simulink library "hvs_framelib_bevlh_det_emot"  (R2016a)
settings: Solver=ode1  StartTime=0.0  StopTime=Inf  FixedStep=0.001  RelTol=1e-3
undefined symbols (not defined in the file): aux_power_flag, dcdc_effmap, dcdc_effmap_cooltemp_3rdD, dcdc_effmap_cur_2ndD, dcdc_effmap_vlt_1stD
libraries: Electrical_to_Mechanical_gen x6, Electrical_converter x4, Electrical_to_Thermal_gen x2, Electrical_charger x2, Powernet x2, Enrg_conv_El_to_Mec_Bosch x2, ePTO x2, simulink x2
(part 2 of 2)

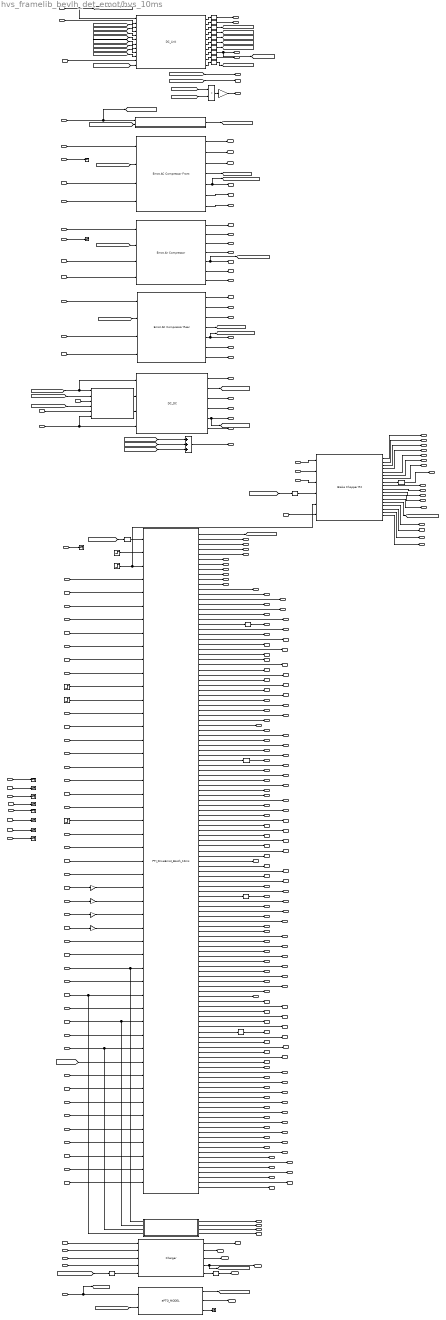
== system hvs_framelib_bevlh_det_emot/hvs_10ms ==
  hvs_dcLink_electricalEnergyStorage_voltage : Inport
  hvs_dcLink_ControllableEnergySource_current : Inport  Port=2
  hvs_dcdcConverter_current : Inport  Port=3
  hvs_driveInverter_coolant_temperature : Inport  Port=4
  hvs_drvEmot1Oil_Temperature : Inport  Port=5
  hvs_brakeResistor_coolant_temperature : Inport  Port=6
  hvs_auxPowerInverter_coolant_temperature : Inport  Port=7
  hvs_inverterAirCompressor_coolant_temperature : Inport  Port=8
  hvs_emot_Emot1_angPos : Inport  Port=9
  hvs_emot_Emot1_angVel : Inport  Port=10
  hvs_emot_Emot1_angAcc : Inport  Port=11
  hvs_emot_Emot2_angAcc : Inport  Port=12
  hvs_emot_Emot2_angPos : Inport  Port=13
  hvs_emot_Emot2_angVel : Inport  Port=14
  hvs_emot_Emot3_angAcc : Inport  Port=15
  hvs_emot_Emot3_angPos : Inport  Port=16
  hvs_emot_Emot3_angVel : Inport  Port=17
  hvs_emot_Emot4_angAcc : Inport  Port=18
  hvs_emot_Emot4_angPos : Inport  Port=19
  hvs_emot_Emot4_angVel : Inport  Port=20
  hvs_emot_AirCompressor_torque : Inport  Port=21
  brc_ControlMode : Inport  Port=22
  brc_PowerReqCh1_kW : Inport  Port=23
  brc_PowerReqCh2_kW : Inport  Port=24
  edcu_EMD1_CMD_ClearErrors : Inport  Port=25
  edcu_EMD1_CMD_ControlMode : Inport  Port=26
  edcu_EMD1_CMD_SpeedRefLim : Inport  Port=27
  pti_tqDesired_PTI1 : Inport  Port=28
  edcu_EMD4_CMD_ClearErrors : Inport  Port=29
  edcu_EMD4_CMD_ControlMode : Inport  Port=30
  edcu_EMD4_CMD_SpeedRefLim : Inport  Port=31
  pti_tqDesired_PTI4 : Inport  Port=32
  vccu_PlugChrg_Stat : Inport  Port=33
  vccu_Pwr_ChargSysSoll : Inport  Port=34
  vccu_TestPwrSLQ_Out : Inport  Port=35
  vccu_CAN_MaxPlginChrgPwrLim : Inport  Port=36
  hvs_emot_AirCondFrontHV_torque : Inport  Port=37
  hvs_emot_AirCondRearHV_torque : Inport  Port=38
  hvsAux_InverterAirCompressor_torque_Rq : Inport  Port=39
  hvsAux_InverterAirCompressor_Voltage_Rq : Inport  Port=40
  hvsAux_InverterAcCompressorFront_torque_Rq : Inport  Port=41
  hvsAux_InverterAcCompressorFront_Voltage_Rq : Inport  Port=42
  hvsAux_InverterAcCompressorRear_torque_Rq : Inport  Port=43
  hvsAux_InverterAcCompressorRear_Voltage_Rq : Inport  Port=44
  hvsAux_dcdcConverter_LvVoltage_Rq : Inport  Port=45
  env_dcLink_aux_power : Inport  Port=46
  edcu_EMD2_CMD_ClearErrors : Inport  Port=47
  edcu_EMD2_CMD_ControlMode : Inport  Port=48
  edcu_EMD2_CMD_SpeedRefLim : Inport  Port=49
  pti_tqDesired_PTI2 : Inport  Port=50
  edcu_EMD3_CMD_ClearErrors : Inport  Port=51
  edcu_EMD3_CMD_ControlMode : Inport  Port=52
  edcu_EMD3_CMD_SpeedRefLim : Inport  Port=53
  pti_tqDesired_PTI3 : Inport  Port=54
  hvs_DCBoxCoolant_Temperature : Inport  Port=55
  hvs_coolHV_current : Inport  Port=56
  env_Temperature : Inport  Port=57
  hvs_drvEmotCoolant_Temperature : Inport  Port=58
  hvs_drvEmot4Oil_Temperature : Inport  Port=59
  hvs_drvEmot2Oil_Temperature : Inport  Port=60
  hvs_drvEmot3Oil_Temperature : Inport  Port=61
  hvs_drvEmot1Coolant_Temperature : Inport  Port=62
  hvs_drvEmot2Coolant_Temperature : Inport  Port=63
  hvs_drvEmot3Coolant_Temperature : Inport  Port=64
  hvs_drvEmot4Coolant_Temperature : Inport  Port=65
  pti_frqSwt_PTI1 : Inport  Port=66
  pti_frqSwt_PTI2 : Inport  Port=67
  pti_frqSwt_PTI3 : Inport  Port=68
  pti_frqSwt_PTI4 : Inport  Port=69
  hvs_drvEmot1CoolantFlow_vdot : Inport  Port=70
  hvs_drvEmot1OilFlow_vdot : Inport  Port=71
  hvs_driveInverterCoolantFlow_vdot : Inport  Port=72
  hvs_drvEmot4CoolantFlow_vdot : Inport  Port=73
  hvs_drvEmot4OilFlow_vdot : Inport  Port=74
  hvs_drvEmot2CoolantFlow_vdot : Inport  Port=75
  hvs_drvEmot2OilFlow_vdot : Inport  Port=76
  hvs_drvEmot3CoolantFlow_vdot : Inport  Port=77
  hvs_drvEmot3OilFlow_vdot : Inport  Port=78
  Brake Chopper RX1 : Electrical_to_Thermal_gen/Brake Chopper RX
  Charger : Electrical_charger/Charger
  DC_DC : Electrical_converter/DC_DC
  DC_Link : Powernet/DC_Link
  EDCU_Dig_SafetyCutOffDG1 : Step  Time=0.812
  Emot AC Compressor Front Generic : Electrical_to_Mechanical_gen/Emot AC Compressor Front
  Emot AC Compressor Rear Generic : Electrical_to_Mechanical_gen/Emot AC Compressor Rear
  Emot Air Compressor Generic : Electrical_to_Mechanical_gen/Emot Air Compressor
  Gain7 : Gain  Gain=1/1000
  HVFreigabeHW1_SiRelay_D : Step  Time=5.502
  HVFreigabeHW2_SiRelay_D : Step  Time=5.502
  HVFreigabeHW3_SiRelay_D : Step  Time=5.502
  HVFreigabeHW4_SiRelay_D : Step  Time=5.502
  PTI_DriveEmot_Bosch_10ms : Enrg_conv_El_to_Mec_Bosch/PTI_DriveEmot_Bosch_10ms
  Process : Subsystem
  Product2 : Product  Inputs=**  RndMeth=Zero
  Rename_Signals_for_PTI_detailed : Subsystem
  Reshape{,1..18} (19 alike) : Reshape
  Sum8 : Sum  Inputs=+++  SaturateOnIntegerOverflow=on  InputSameDT=on  OutDataTypeStr=Inherit: Same as first input
  Terminator{,1..10,15} (12 alike) : Terminator
  ePTO_MODEL : ePTO/ePTO_MODEL
  rad/sectorpm{,1..3} (4 alike) : Gain  Gain=30/pi
  sub_env_aux : Subsystem
  hvs_dcLink_electricalEnergyStorage_current : Outport
  hvs_dcLink_ControllableEnergySource_voltage : Outport  Port=2
  hvs_dcdcConverter_voltage : Outport  Port=3
  hvs_driveInverter_wasteHeat_power : Outport  Port=4
  hvs_drvEmotWasteHeat_power : Outport  Port=5
  hvs_drvEmot1WasteHeat_power : Outport  Port=6
  hvs_drvEmot2WasteHeat_power : Outport  Port=7
  hvs_drvEmot3WasteHeat_power : Outport  Port=8
  hvs_drvEmot4WasteHeat_power : Outport  Port=9
  hvs_brakeResistor_wasteHeat_power : Outport  Port=10
  hvs_auxPowerInverter_wasteHeat_power : Outport  Port=11
  hvs_inverterAirCompressor_wasteHeat_power : Outport  Port=12
  hvs_emot_Emot1_torque : Outport  Port=13
  hvs_emot_Emot2_torque : Outport  Port=14
  hvs_emot_Emot3_torque : Outport  Port=15
  hvs_emot_Emot4_torque : Outport  Port=16
  hvs_emot_AirCompressor_angAcc : Outport  Port=17
  hvs_emot_AirCompressor_angPos : Outport  Port=18
  hvs_emot_AirCompressor_angVel : Outport  Port=19
  hvs_emot_AirCondFrontHV_angAcc : Outport  Port=20
  hvs_emot_AirCondFrontHV_angPos : Outport  Port=21
  hvs_emot_AirCondFrontHV_angVel : Outport  Port=22
  hvs_emot_AirCondRearHV_angAcc : Outport  Port=23
  hvs_emot_AirCondRearHV_angVel : Outport  Port=24
  hvs_emot_AirCondRearHV_angPos : Outport  Port=25
  hvs_BRC_ACT_DigitalInput1 : Outport  Port=26
  hvs_BRC_ACT_InverterState : Outport  Port=27
  hvs_BRC_ACT_MaxAvailablePowerCh1 : Outport  Port=28
  hvs_BRC_ACT_MaxAvailablePowerCh1_VAL : Outport  Port=29
  hvs_BRC_ACT_PowerCh1 : Outport  Port=30
  hvs_BRC_ACT_MaxAvailablePowerCh2 : Outport  Port=31
  hvs_BRC_ACT_PowerCh2 : Outport  Port=32
  hvs_BRC_ACT_DcLinkVoltage : Outport  Port=33
  hvs_BRC_ACT_ExtTemperatureCh1 : Outport  Port=34
  hvs_BRC_ACT_ExtTemperatureCh2 : Outport  Port=35
  hvs_BRC_ACT_JunctionTempCh1 : Outport  Port=36
  hvs_BRC_ACT_JunctionTempCh2 : Outport  Port=37
  hvs_EMD1_ACT_DigitalInput1 : Outport  Port=38
  hvs_EMD1_ACT_InverterState : Outport  Port=39
  hvs_EMD1_ACT_MaxAvailableTorque : Outport  Port=40
  hvs_EMD1_ACT_ReferenceTorqueLim : Outport  Port=41
  hvs_EMD1_ACT_Torque : Outport  Port=42
  hvs_EMD1_ACT_DcLinkPower : Outport  Port=43
  hvs_EMD1_ACT_MotorSpeed : Outport  Port=44
  hvs_EMD1_ACT_DcLinkVoltage : Outport  Port=45
  hvs_EMD1_ACT_MaxJunctionTemp : Outport  Port=46
  hvs_EMD1_ACT_MotorTemperature : Outport  Port=47
  hvs_EMD1_ACT_RotorTemperature : Outport  Port=48
  hvs_EMD1_ACT_InverterLosses : Outport  Port=49
  hvs_EMD1_ACT_MotorLosses : Outport  Port=50
  hvs_EMD1_uStator : Outport  Port=51
  hvs_EMD1_iStator : Outport  Port=52
  hvs_EMD1_modIdx : Outport  Port=53
  hvs_EMD1_cosPhi : Outport  Port=54
  hvs_EMD1_ACT_tSnsrPwrModlMax : Outport  Port=55
  hvs_EMD1_ACT_tCapSnsr : Outport  Port=56
  hvs_EMD1_ACT_tCapCoil : Outport  Port=57
  hvs_EMD1_ACT_tCapAcCnctr : Outport  Port=58
  hvs_EMD1_ACT_tCapDcCnctr : Outport  Port=59
  hvs_EMD1_ACT_tIvtrAcRail : Outport  Port=60
  hvs_EMD1_ACT_tIvtrDcRail : Outport  Port=61
  hvs_EMD1_ACT_tIvtrAcRailIphaSnsr : Outport  Port=62
  hvs_EMD1_ACT_tIvtrDcRailCnctr : Outport  Port=63
  hvs_EMD1_ACT_tCoolIvtrOuttk : Outport  Port=64
  hvs_EMD1_ACT_tCoolantIvtrIntk : Outport  Port=65
  hvs_EMD4_ACT_DigitalInput1 : Outport  Port=66
  hvs_EMD4_ACT_InverterState : Outport  Port=67
  hvs_EMD4_ACT_MaxAvailableTorque : Outport  Port=68
  hvs_EMD4_ACT_ReferenceTorqueLim : Outport  Port=69
  hvs_EMD4_ACT_Torque : Outport  Port=70
  hvs_EMD4_ACT_DcLinkPower : Outport  Port=71
  hvs_EMD4_ACT_MotorSpeed : Outport  Port=72
  hvs_EMD4_ACT_DcLinkVoltage : Outport  Port=73
  hvs_EMD4_ACT_MaxJunctionTemperature : Outport  Port=74
  hvs_EMD4_ACT_MotorTemperature : Outport  Port=75
  hvs_EMD4_ACT_RotorTemperature : Outport  Port=76
  hvs_EMD4_ACT_InverterLosses : Outport  Port=77
  hvs_EMD4_ACT_MotorLosses : Outport  Port=78
  hvs_EMD4_uStator : Outport  Port=79
  hvs_EMD4_iStator : Outport  Port=80
  hvs_EMD4_modIdx : Outport  Port=81
  hvs_EMD4_cosPhi : Outport  Port=82
  hvs_EMD4_ACT_tSnsrPwrModlMax : Outport  Port=83
  hvs_EMD4_ACT_tCapSnsr : Outport  Port=84
  hvs_EMD4_ACT_tCapCoil : Outport  Port=85
  hvs_EMD4_ACT_tCapAcCnctr : Outport  Port=86
  hvs_EMD4_ACT_tCapDcCnctr : Outport  Port=87
  hvs_EMD4_ACT_tIvtrAcRail : Outport  Port=88
  hvs_EMD4_ACT_tIvtrDcRail : Outport  Port=89
  hvs_EMD4_ACT_tIvtrAcRailIphaSnsr : Outport  Port=90
  hvs_EMD4_ACT_tIvtrDcRailCnctr : Outport  Port=91
  hvs_EMD4_ACT_tCoolIvtrOuttk : Outport  Port=92
  hvs_EMD4_ACT_tCoolantIvtrIntk : Outport  Port=93
  hvs_EMD3_ACT_DigitalInput1 : Outport  Port=94
  hvs_EMD3_ACT_InverterState : Outport  Port=95
  hvs_EMD3_ACT_MaxAvailableTorque : Outport  Port=96
  hvs_EMD3_ACT_ReferenceTorqueLim : Outport  Port=97
  hvs_EMD3_ACT_Torque : Outport  Port=98
  hvs_EMD3_ACT_DcLinkPower : Outport  Port=99
  hvs_EMD3_ACT_MotorSpeed : Outport  Port=100
  hvs_EMD3_ACT_DcLinkVoltage : Outport  Port=101
  hvs_EMD3_ACT_MaxJunctionTemp : Outport  Port=102
  hvs_EMD3_ACT_MotorTemperature : Outport  Port=103
  hvs_EMD3_ACT_RotorTemperature : Outport  Port=104
  hvs_EMD3_ACT_InverterLosses : Outport  Port=105
  hvs_EMD3_ACT_MotorLosses : Outport  Port=106
  hvs_EMD3_uStator : Outport  Port=107
  hvs_EMD3_iStator : Outport  Port=108
  hvs_EMD3_modIdx : Outport  Port=109
  hvs_EMD3_cosPhi : Outport  Port=110
  hvs_EMD3_ACT_tSnsrPwrModlMax : Outport  Port=111
  hvs_EMD3_ACT_tCapSnsr : Outport  Port=112
  hvs_EMD3_ACT_tCapCoil : Outport  Port=113
  hvs_EMD3_ACT_tCapAcCnctr : Outport  Port=114
  hvs_EMD3_ACT_tCapDcCnctr : Outport  Port=115
  hvs_EMD3_ACT_tIvtrAcRail : Outport  Port=116
  hvs_EMD3_ACT_tIvtrDcRail : Outport  Port=117
  hvs_EMD3_ACT_tIvtrAcRailIphaSnsr : Outport  Port=118
  hvs_EMD3_ACT_tIvtrDcRailCnctr : Outport  Port=119
  hvs_EMD3_ACT_tCoolIvtrOuttk : Outport  Port=120
  hvs_EMD3_ACT_tCoolantIvtrIntk : Outport  Port=121
  hvs_EMD2_ACT_DigitalInput1 : Outport  Port=122
  hvs_EMD2_ACT_InverterState : Outport  Port=123
  hvs_EMD2_ACT_MaxAvailableTorque : Outport  Port=124
  hvs_EMD2_ACT_ReferenceTorqueLim : Outport  Port=125
  hvs_EMD2_ACT_Torque : Outport  Port=126
  hvs_EMD2_ACT_DcLinkPower : Outport  Port=127
  hvs_EMD2_ACT_MotorSpeed : Outport  Port=128
  hvs_EMD2_ACT_DcLinkVoltage : Outport  Port=129
  hvs_EMD2_ACT_MaxJunctionTemp : Outport  Port=130
  hvs_EMD2_ACT_MotorTemperature : Outport  Port=131
  hvs_EMD2_ACT_RotorTemperature : Outport  Port=132
  hvs_EMD2_ACT_InverterLosses : Outport  Port=133
  hvs_EMD2_ACT_MotorLosses : Outport  Port=134
  hvs_EMD2_uStator : Outport  Port=135
  hvs_EMD2_iStator : Outport  Port=136
  hvs_EMD2_modIdx : Outport  Port=137
  hvs_EMD2_cosPhi : Outport  Port=138
  hvs_EMD2_ACT_tSnsrPwrModlMax : Outport  Port=139
  hvs_EMD2_ACT_tCapSnsr : Outport  Port=140
  hvs_EMD2_ACT_tCapCoil : Outport  Port=141
  hvs_EMD2_ACT_tCapAcCnctr : Outport  Port=142
  hvs_EMD2_ACT_tCapDcCnctr : Outport  Port=143
  hvs_EMD2_ACT_tIvtrAcRail : Outport  Port=144
  hvs_EMD2_ACT_tIvtrDcRail : Outport  Port=145
  hvs_EMD2_ACT_tIvtrAcRailIphaSnsr : Outport  Port=146
  hvs_EMD2_ACT_tIvtrDcRailCnctr : Outport  Port=147
  hvs_EMD2_ACT_tCoolIvtrOuttk : Outport  Port=148
  hvs_EMD2_ACT_tCoolantIvtrIntk : Outport  Port=149
  hvs_charger_pwrChrgPhy : Outport  Port=150
  hvs_charger_ExtChrgr_Isolation_ResistanceCval : Outport  Port=151
  hvs_VCCU_DCLInk_vlt : Outport  Port=152
  hvs_InverterAirCompressor_hvCurrent : Outport  Port=153
  hvs_InverterAirCompressor_hvVoltage : Outport  Port=154
  hvs_emot_AirCompressor_nEmot : Outport  Port=155
  hvs_InverterAcCompressor_hvCurrent : Outport  Port=156
  hvs_InverterAcCompressor_hvVoltage : Outport  Port=157
  hvs_emot_AcCompressor_nEmot : Outport  Port=158
  hvs_InverterAcCompressorRear_hvCurrent : Outport  Port=159
  hvs_InverterAcCompressorRear_hvVoltage : Outport  Port=160
  hvs_emot_AcCompressorRear_nEmot : Outport  Port=161
  hvs_dcdcConverter_HvVoltage : Outport  Port=162
  hvs_dcdcConverter_LvVoltage : Outport  Port=163
  hvs_dcdcConverter_HvCurrent : Outport  Port=164
  hvs_dcdcConverter_LvCurrent : Outport  Port=165
  hvs_dcLink_aux_current : Outport  Port=166
  hvs_DCBoxWasteHeat_power : Outport  Port=167
  hvs_coolHV_voltage : Outport  Port=168
  hvs_ePTO_Elec_Power : Outport  Port=169
  hvs_charger_current : Outport  Port=170
  hvs_dcLink_drive_emot_current : Outport  Port=171
  hvs_dcLink_BrakeResistor_current : Outport  Port=172
  hvs_dcLink_aux_Power : Outport  Port=173
  hvs_EMD2_ACT_Torque_Nm : Outport  Port=174
  hvs_EMD3_ACT_Torque_Nm : Outport  Port=175
  hvs_EMD1_ACT_Torque_Nm : Outport  Port=176
  hvs_EMD4_ACT_Torque_Nm : Outport  Port=177
  hvs_drvEmot2WasteHeatcoolant_power : Outport  Port=178
  hvs_drvEmot2WasteHeatoil_power : Outport  Port=179
  hvs_drvEmot3WasteHeatcoolant_power : Outport  Port=180
  hvs_drvEmot3WasteHeatoil_power : Outport  Port=181
  hvs_drvEmot1WasteHeatcoolant_power : Outport  Port=182
  hvs_drvEmot1WasteHeatoil_power : Outport  Port=183
  hvs_drvEmot4WasteHeatcoolant_power : Outport  Port=184
  hvs_drvEmot4WasteHeatoil_power : Outport  Port=185
  hvs_BRC_ACT_MaxAvailablePowerCh1_kW : Outport  Port=186
  hvs_BRC_ACT_PowerCh1_kW : Outport  Port=187
  hvs_BRC_ACT_MaxAvailablePowerCh2_kW : Outport  Port=188
  hvs_BRC_ACT_PowerCh2_kW : Outport  Port=189
  wires:
  [hvs_dcLink_aux_current] -> Product2/1
  [hvs_APIs_DCLink_vlt] -> Product2/2
  Product2/1 -> Gain7/1
  Gain7/1 -> hvs_dcLink_aux_Power/1
  Rename_Signals_for_PTI_detailed/1(hvs_EMD1_ACT_tCoolantIvtrIntk) -> hvs_EMD1_ACT_tCoolantIvtrIntk/1
  Rename_Signals_for_PTI_detailed/4(hvs_EMD4_ACT_tCoolantIvtrIntk) -> hvs_EMD4_ACT_tCoolantIvtrIntk/1
  Rename_Signals_for_PTI_detailed/3(hvs_EMD3_ACT_tCoolantIvtrIntk) -> hvs_EMD3_ACT_tCoolantIvtrIntk/1
  Rename_Signals_for_PTI_detailed/2(hvs_EMD2_ACT_tCoolantIvtrIntk) -> hvs_EMD2_ACT_tCoolantIvtrIntk/1
  hvs_drvEmot2Coolant_Temperature/1 -> Rename_Signals_for_PTI_detailed/2(hvs_drvEmot2Coolant_Temperature), PTI_DriveEmot_Bosch_10ms/37
  PTI_DriveEmot_Bosch_10ms/27 -> hvs_EMD1_modIdx/1
  PTI_DriveEmot_Bosch_10ms/28 -> hvs_EMD1_cosPhi/1
  PTI_DriveEmot_Bosch_10ms/38 -> hvs_EMD1_ACT_tCoolIvtrOuttk/1
  PTI_DriveEmot_Bosch_10ms/37 -> hvs_EMD1_ACT_tIvtrDcRailCnctr/1
  PTI_DriveEmot_Bosch_10ms/36 -> hvs_EMD1_ACT_tIvtrAcRailIphaSnsr/1
  PTI_DriveEmot_Bosch_10ms/35 -> hvs_EMD1_ACT_tIvtrDcRail/1
  PTI_DriveEmot_Bosch_10ms/34 -> hvs_EMD1_ACT_tIvtrAcRail/1
  PTI_DriveEmot_Bosch_10ms/33 -> hvs_EMD1_ACT_tCapDcCnctr/1
  PTI_DriveEmot_Bosch_10ms/32 -> hvs_EMD1_ACT_tCapAcCnctr/1
  PTI_DriveEmot_Bosch_10ms/31 -> hvs_EMD1_ACT_tCapCoil/1
  PTI_DriveEmot_Bosch_10ms/29 -> hvs_EMD1_ACT_tSnsrPwrModlMax/1
  PTI_DriveEmot_Bosch_10ms/30 -> hvs_EMD1_ACT_tCapSnsr/1
  PTI_DriveEmot_Bosch_10ms/53 -> hvs_EMD4_iStator/1
  PTI_DriveEmot_Bosch_10ms/52 -> hvs_EMD4_uStator/1
  PTI_DriveEmot_Bosch_10ms/51 -> hvs_EMD4_ACT_MotorLosses/1
  PTI_DriveEmot_Bosch_10ms/50 -> hvs_EMD4_ACT_InverterLosses/1
  PTI_DriveEmot_Bosch_10ms/49 -> hvs_EMD4_ACT_RotorTemperature/1
  PTI_DriveEmot_Bosch_10ms/48 -> hvs_EMD4_ACT_MotorTemperature/1
  PTI_DriveEmot_Bosch_10ms/47 -> hvs_EMD4_ACT_MaxJunctionTemperature/1
  PTI_DriveEmot_Bosch_10ms/46 -> Reshape10/1
  PTI_DriveEmot_Bosch_10ms/45 -> hvs_EMD4_ACT_MotorSpeed/1
  PTI_DriveEmot_Bosch_10ms/44 -> hvs_EMD4_ACT_DcLinkPower/1
  PTI_DriveEmot_Bosch_10ms/43 -> hvs_EMD4_ACT_Torque/1
  PTI_DriveEmot_Bosch_10ms/42 -> hvs_EMD4_ACT_ReferenceTorqueLim/1
  PTI_DriveEmot_Bosch_10ms/41 -> hvs_EMD4_ACT_MaxAvailableTorque/1
  PTI_DriveEmot_Bosch_10ms/40 -> hvs_EMD4_ACT_InverterState/1
  PTI_DriveEmot_Bosch_10ms/39 -> hvs_EMD4_ACT_DigitalInput1/1
  PTI_DriveEmot_Bosch_10ms/54 -> hvs_EMD4_modIdx/1
  PTI_DriveEmot_Bosch_10ms/55 -> hvs_EMD4_cosPhi/1
  PTI_DriveEmot_Bosch_10ms/58 -> hvs_EMD4_ACT_tCapCoil/1
  PTI_DriveEmot_Bosch_10ms/59 -> hvs_EMD4_ACT_tCapAcCnctr/1
  PTI_DriveEmot_Bosch_10ms/60 -> hvs_EMD4_ACT_tCapDcCnctr/1
  PTI_DriveEmot_Bosch_10ms/61 -> hvs_EMD4_ACT_tIvtrAcRail/1
  PTI_DriveEmot_Bosch_10ms/62 -> hvs_EMD4_ACT_tIvtrDcRail/1
  PTI_DriveEmot_Bosch_10ms/63 -> hvs_EMD4_ACT_tIvtrAcRailIphaSnsr/1
  PTI_DriveEmot_Bosch_10ms/64 -> hvs_EMD4_ACT_tIvtrDcRailCnctr/1
  PTI_DriveEmot_Bosch_10ms/65 -> hvs_EMD4_ACT_tCoolIvtrOuttk/1
  PTI_DriveEmot_Bosch_10ms/56 -> hvs_EMD4_ACT_tSnsrPwrModlMax/1
  PTI_DriveEmot_Bosch_10ms/57 -> hvs_EMD4_ACT_tCapSnsr/1
  PTI_DriveEmot_Bosch_10ms/80 -> hvs_EMD3_iStator/1
  PTI_DriveEmot_Bosch_10ms/79 -> hvs_EMD3_uStator/1
  PTI_DriveEmot_Bosch_10ms/78 -> hvs_EMD3_ACT_MotorLosses/1
  PTI_DriveEmot_Bosch_10ms/77 -> hvs_EMD3_ACT_InverterLosses/1
  PTI_DriveEmot_Bosch_10ms/76 -> hvs_EMD3_ACT_RotorTemperature/1
  PTI_DriveEmot_Bosch_10ms/75 -> hvs_EMD3_ACT_MotorTemperature/1
  PTI_DriveEmot_Bosch_10ms/74 -> hvs_EMD3_ACT_MaxJunctionTemp/1
  PTI_DriveEmot_Bosch_10ms/73 -> Reshape13/1
  PTI_DriveEmot_Bosch_10ms/72 -> hvs_EMD3_ACT_MotorSpeed/1
  PTI_DriveEmot_Bosch_10ms/71 -> hvs_EMD3_ACT_DcLinkPower/1
  PTI_DriveEmot_Bosch_10ms/70 -> hvs_EMD3_ACT_Torque/1
  PTI_DriveEmot_Bosch_10ms/69 -> hvs_EMD3_ACT_ReferenceTorqueLim/1
  PTI_DriveEmot_Bosch_10ms/68 -> hvs_EMD3_ACT_MaxAvailableTorque/1
  PTI_DriveEmot_Bosch_10ms/67 -> hvs_EMD3_ACT_InverterState/1
  PTI_DriveEmot_Bosch_10ms/66 -> hvs_EMD3_ACT_DigitalInput1/1
  PTI_DriveEmot_Bosch_10ms/81 -> hvs_EMD3_modIdx/1
  PTI_DriveEmot_Bosch_10ms/82 -> hvs_EMD3_cosPhi/1
  PTI_DriveEmot_Bosch_10ms/83 -> hvs_EMD3_ACT_tSnsrPwrModlMax/1
  PTI_DriveEmot_Bosch_10ms/84 -> hvs_EMD3_ACT_tCapSnsr/1
  PTI_DriveEmot_Bosch_10ms/85 -> hvs_EMD3_ACT_tCapCoil/1
  PTI_DriveEmot_Bosch_10ms/86 -> hvs_EMD3_ACT_tCapAcCnctr/1
  PTI_DriveEmot_Bosch_10ms/87 -> hvs_EMD3_ACT_tCapDcCnctr/1
  PTI_DriveEmot_Bosch_10ms/88 -> hvs_EMD3_ACT_tIvtrAcRail/1
  PTI_DriveEmot_Bosch_10ms/89 -> hvs_EMD3_ACT_tIvtrDcRail/1
  PTI_DriveEmot_Bosch_10ms/90 -> hvs_EMD3_ACT_tIvtrAcRailIphaSnsr/1
  PTI_DriveEmot_Bosch_10ms/91 -> hvs_EMD3_ACT_tIvtrDcRailCnctr/1
  PTI_DriveEmot_Bosch_10ms/92 -> hvs_EMD3_ACT_tCoolIvtrOuttk/1
  PTI_DriveEmot_Bosch_10ms/108 -> hvs_EMD2_modIdx/1
  PTI_DriveEmot_Bosch_10ms/109 -> hvs_EMD2_cosPhi/1
  PTI_DriveEmot_Bosch_10ms/119 -> hvs_EMD2_ACT_tCoolIvtrOuttk/1
  PTI_DriveEmot_Bosch_10ms/118 -> hvs_EMD2_ACT_tIvtrDcRailCnctr/1
  PTI_DriveEmot_Bosch_10ms/117 -> hvs_EMD2_ACT_tIvtrAcRailIphaSnsr/1
  PTI_DriveEmot_Bosch_10ms/116 -> hvs_EMD2_ACT_tIvtrDcRail/1
  PTI_DriveEmot_Bosch_10ms/115 -> hvs_EMD2_ACT_tIvtrAcRail/1
  PTI_DriveEmot_Bosch_10ms/114 -> hvs_EMD2_ACT_tCapDcCnctr/1
  PTI_DriveEmot_Bosch_10ms/113 -> hvs_EMD2_ACT_tCapAcCnctr/1
  PTI_DriveEmot_Bosch_10ms/112 -> hvs_EMD2_ACT_tCapCoil/1
  PTI_DriveEmot_Bosch_10ms/111 -> hvs_EMD2_ACT_tCapSnsr/1
  PTI_DriveEmot_Bosch_10ms/110 -> hvs_EMD2_ACT_tSnsrPwrModlMax/1
  Reshape18/1 -> hvs_EMD2_ACT_DcLinkVoltage/1
  PTI_DriveEmot_Bosch_10ms/107 -> hvs_EMD2_iStator/1
  PTI_DriveEmot_Bosch_10ms/106 -> hvs_EMD2_uStator/1
  PTI_DriveEmot_Bosch_10ms/105 -> hvs_EMD2_ACT_MotorLosses/1
  PTI_DriveEmot_Bosch_10ms/104 -> hvs_EMD2_ACT_InverterLosses/1
  PTI_DriveEmot_Bosch_10ms/103 -> hvs_EMD2_ACT_RotorTemperature/1
  PTI_DriveEmot_Bosch_10ms/102 -> hvs_EMD2_ACT_MotorTemperature/1
  PTI_DriveEmot_Bosch_10ms/101 -> hvs_EMD2_ACT_MaxJunctionTemp/1
  PTI_DriveEmot_Bosch_10ms/100 -> Reshape18/1
  PTI_DriveEmot_Bosch_10ms/99 -> hvs_EMD2_ACT_MotorSpeed/1
  PTI_DriveEmot_Bosch_10ms/98 -> hvs_EMD2_ACT_DcLinkPower/1
  PTI_DriveEmot_Bosch_10ms/97 -> hvs_EMD2_ACT_Torque/1
  PTI_DriveEmot_Bosch_10ms/96 -> hvs_EMD2_ACT_ReferenceTorqueLim/1
  PTI_DriveEmot_Bosch_10ms/95 -> hvs_EMD2_ACT_MaxAvailableTorque/1
  PTI_DriveEmot_Bosch_10ms/94 -> hvs_EMD2_ACT_InverterState/1
  PTI_DriveEmot_Bosch_10ms/93 -> hvs_EMD2_ACT_DigitalInput1/1
  PTI_DriveEmot_Bosch_10ms/26 -> hvs_EMD1_iStator/1
  PTI_DriveEmot_Bosch_10ms/25 -> hvs_EMD1_uStator/1
  PTI_DriveEmot_Bosch_10ms/22 -> hvs_EMD1_ACT_RotorTemperature/1
  PTI_DriveEmot_Bosch_10ms/24 -> hvs_EMD1_ACT_MotorLosses/1
  PTI_DriveEmot_Bosch_10ms/23 -> hvs_EMD1_ACT_InverterLosses/1
  pti_frqSwt_PTI1/1 -> PTI_DriveEmot_Bosch_10ms/23
  EDCU_Dig_SafetyCutOffDG1/1 -> PTI_DriveEmot_Bosch_10ms/22
  pti_tqDesired_PTI3/1 -> PTI_DriveEmot_Bosch_10ms/21
  edcu_EMD3_CMD_SpeedRefLim/1 -> PTI_DriveEmot_Bosch_10ms/20
  edcu_EMD3_CMD_ControlMode/1 -> PTI_DriveEmot_Bosch_10ms/19
  edcu_EMD3_CMD_ClearErrors/1 -> PTI_DriveEmot_Bosch_10ms/18
  pti_tqDesired_PTI2/1 -> PTI_DriveEmot_Bosch_10ms/17
  edcu_EMD2_CMD_SpeedRefLim/1 -> PTI_DriveEmot_Bosch_10ms/16
  edcu_EMD2_CMD_ControlMode/1 -> PTI_DriveEmot_Bosch_10ms/15
  edcu_EMD2_CMD_ClearErrors/1 -> PTI_DriveEmot_Bosch_10ms/14
  HVFreigabeHW3_SiRelay_D/1 -> PTI_DriveEmot_Bosch_10ms/13
  HVFreigabeHW2_SiRelay_D/1 -> PTI_DriveEmot_Bosch_10ms/12
  pti_tqDesired_PTI1/1 -> PTI_DriveEmot_Bosch_10ms/7
  hvs_emot_Emot1_angAcc/1 -> Terminator15/1
  hvs_coolHV_current/1 -> DC_Link/11
  Reshape16/1 -> hvs_coolHV_voltage/1
  DC_Link/9 -> Reshape16/1
  Reshape15/1 -> hvs_dcLink_aux_current/1, [hvs_dcLink_aux_current]
  Reshape14/1 -> hvs_dcLink_ControllableEnergySource_voltage/1
  Reshape13/1 -> hvs_EMD3_ACT_DcLinkVoltage/1
  PTI_DriveEmot_Bosch_10ms/18 -> hvs_EMD1_ACT_MotorSpeed/1
  Reshape9/1 -> hvs_EMD1_ACT_DcLinkVoltage/1
  PTI_DriveEmot_Bosch_10ms/17 -> hvs_EMD1_ACT_DcLinkPower/1
  PTI_DriveEmot_Bosch_10ms/16 -> hvs_EMD1_ACT_Torque/1
  PTI_DriveEmot_Bosch_10ms/15 -> hvs_EMD1_ACT_ReferenceTorqueLim/1
  PTI_DriveEmot_Bosch_10ms/14 -> hvs_EMD1_ACT_MaxAvailableTorque/1
  PTI_DriveEmot_Bosch_10ms/13 -> hvs_EMD1_ACT_InverterState/1
  PTI_DriveEmot_Bosch_10ms/7 -> hvs_drvEmotWasteHeat_power/1
  PTI_DriveEmot_Bosch_10ms/6 -> hvs_driveInverter_wasteHeat_power/1
  PTI_DriveEmot_Bosch_10ms/2 -> hvs_emot_Emot1_torque/1
  [hvs_InverterAcCompressorRear_hvCurrent] -> DC_Link/9
  [hvs_InverterAcCompressor_hvCurrent] -> DC_Link/8
  Emot AC Compressor Front Generic/5 -> [hvs_InverterAcCompressor_hvCurrent], hvs_InverterAcCompressor_hvCurrent/1
  Charger/5 -> Reshape12/1
  DC_Link/6 -> Reshape4/1
  [hvs_dcLink_charger_current] -> DC_Link/7
  Charger/4 -> hvs_charger_current/1, [hvs_dcLink_charger_current]
  Charger/3 -> hvs_charger_ExtChrgr_Isolation_ResistanceCval/1
  Charger/2 -> hvs_charger_pwrChrgPhy/1
  vccu_PlugChrg_Stat/1 -> Charger/1
  vccu_Pwr_ChargSysSoll/1 -> Charger/2
  vccu_TestPwrSLQ_Out/1 -> Charger/3
  [hvs_charger_DCLink_vlt] -> Reshape11/1
  vccu_CAN_MaxPlginChrgPwrLim/1 -> Charger/4
  pti_tqDesired_PTI4/1 -> PTI_DriveEmot_Bosch_10ms/11
  edcu_EMD4_CMD_SpeedRefLim/1 -> PTI_DriveEmot_Bosch_10ms/10
  edcu_EMD4_CMD_ControlMode/1 -> PTI_DriveEmot_Bosch_10ms/9
  edcu_EMD4_CMD_ClearErrors/1 -> PTI_DriveEmot_Bosch_10ms/8
  edcu_EMD1_CMD_SpeedRefLim/1 -> PTI_DriveEmot_Bosch_10ms/6
  edcu_EMD1_CMD_ControlMode/1 -> PTI_DriveEmot_Bosch_10ms/5
  edcu_EMD1_CMD_ClearErrors/1 -> PTI_DriveEmot_Bosch_10ms/4
  PTI_DriveEmot_Bosch_10ms/21 -> hvs_EMD1_ACT_MotorTemperature/1
  PTI_DriveEmot_Bosch_10ms/20 -> hvs_EMD1_ACT_MaxJunctionTemp/1
  PTI_DriveEmot_Bosch_10ms/19 -> Reshape9/1
  PTI_DriveEmot_Bosch_10ms/3 -> hvs_emot_Emot2_torque/1
  hvs_emot_Emot2_angVel/1 -> rad/sectorpm1/1
  hvs_emot_Emot2_angPos/1 -> Terminator3/1
  hvs_emot_Emot2_angAcc/1 -> Terminator2/1
  hvs_emot_Emot1_angPos/1 -> Terminator1/1
  HVFreigabeHW1_SiRelay_D/1 -> PTI_DriveEmot_Bosch_10ms/2
  [hvs_dcLink_BrakeResistor_current] -> DC_Link/6
  HVFreigabeHW4_SiRelay_D/1 -> Brake Chopper RX1/5, PTI_DriveEmot_Bosch_10ms/3
  [hvs_emot_AirCompressor_emot_current] -> DC_Link/5
  [hvs_dcLink_drive_emot_current] -> DC_Link/4
  [hvs_inverter_drive_emot_voltage] -> Reshape8/1
  DC_Link/5 -> Reshape3/1
  hvs_emot_Emot1_angVel/1 -> rad/sectorpm/1
  [hvs_inverter_BrakeResistor_voltage] -> Reshape6/1
  DC_Link/4 -> Reshape2/1
  hvs_dcLink_ControllableEnergySource_current/1 -> DC_Link/2
  hvs_dcLink_electricalEnergyStorage_voltage/1 -> DC_Link/1, [hvs_dcLink_electricalEnergyStorage_voltage]
  DC_Link/2 -> Reshape14/1
  DC_Link/1 -> Reshape/1
  hvs_emot_AirCompressor_torque/1 -> Emot Air Compressor Generic/1
  Emot Air Compressor Generic/1 -> hvs_emot_AirCompressor_angAcc/1
  Emot Air Compressor Generic/2 -> hvs_emot_AirCompressor_angPos/1
  Emot Air Compressor Generic/3 -> hvs_emot_AirCompressor_angVel/1
  Emot Air Compressor Generic/4 -> hvs_inverterAirCompressor_wasteHeat_power/1
  Emot Air Compressor Generic/5 -> hvs_InverterAirCompressor_hvCurrent/1, [hvs_emot_AirCompressor_emot_current]
  Emot Air Compressor Generic/7 -> hvs_emot_AirCompressor_nEmot/1
  Emot Air Compressor Generic/6 -> hvs_InverterAirCompressor_hvVoltage/1
  DC_Link/7 -> Reshape5/1
  [hvs_APIs_DCLink_vlt] -> Emot Air Compressor Generic/2
  hvsAux_InverterAirCompressor_torque_Rq/1 -> Emot Air Compressor Generic/3
  hvsAux_InverterAirCompressor_Voltage_Rq/1 -> Emot Air Compressor Generic/4
  hvs_inverterAirCompressor_coolant_temperature/1 -> Terminator/1
  hvs_auxPowerInverter_coolant_temperature/1 -> Terminator5/1
  [hvs_APIs_DCLink_vlt] -> Emot AC Compressor Front Generic/2
  hvs_emot_AirCondFrontHV_torque/1 -> Emot AC Compressor Front Generic/1
  hvsAux_InverterAcCompressorFront_torque_Rq/1 -> Emot AC Compressor Front Generic/3
  hvsAux_InverterAcCompressorFront_Voltage_Rq/1 -> Emot AC Compressor Front Generic/4
  Emot AC Compressor Front Generic/1 -> hvs_emot_AirCondFrontHV_angAcc/1
  Emot AC Compressor Front Generic/2 -> hvs_emot_AirCondFrontHV_angPos/1
  Emot AC Compressor Front Generic/3 -> hvs_emot_AirCondFrontHV_angVel/1
  Emot AC Compressor Front Generic/7 -> hvs_emot_AcCompressor_nEmot/1
  Emot AC Compressor Front Generic/6 -> hvs_InverterAcCompressor_hvVoltage/1
  Emot AC Compressor Front Generic/4 -> [hvs_API1_wasteHeat_power]
  hvs_emot_AirCondRearHV_torque/1 -> Emot AC Compressor Rear Generic/1
  [hvs_APIs_DCLink_vlt] -> Emot AC Compressor Rear Generic/2
  hvsAux_InverterAcCompressorRear_torque_Rq/1 -> Emot AC Compressor Rear Generic/3
  hvsAux_InverterAcCompressorRear_Voltage_Rq/1 -> Emot AC Compressor Rear Generic/4
  Emot AC Compressor Rear Generic/1 -> hvs_emot_AirCondRearHV_angAcc/1
  Emot AC Compressor Rear Generic/3 -> hvs_emot_AirCondRearHV_angVel/1
  Emot AC Compressor Rear Generic/2 -> hvs_emot_AirCondRearHV_angPos/1
  Emot AC Compressor Rear Generic/7 -> hvs_emot_AcCompressorRear_nEmot/1
  Emot AC Compressor Rear Generic/6 -> hvs_InverterAcCompressorRear_hvVoltage/1
  Emot AC Compressor Rear Generic/5 -> hvs_InverterAcCompressorRear_hvCurrent/1, [hvs_InverterAcCompressorRear_hvCurrent]
  Emot AC Compressor Rear Generic/4 -> [hvs_API3_wasteHeat_power]
  [hvs_dcdcConverter_voltage] -> DC_DC/1, Process/1(hvs_dcdcConverter_voltage)  "hvs_dcdcConverter_voltage"
  DC_DC/2 -> [hvs_DCL_wasteHeat_power]
  DC_DC/1 -> hvs_dcdcConverter_voltage/1
  DC_Link/3 -> Reshape1/1
  DC_DC/3 -> hvs_dcdcConverter_HvVoltage/1
  DC_DC/4 -> hvs_dcdcConverter_LvVoltage/1
  DC_DC/5 -> [hvs_dcdc_current], hvs_dcdcConverter_HvCurrent/1
  DC_DC/6 -> hvs_dcdcConverter_LvCurrent/1
  Sum8/1 -> hvs_auxPowerInverter_wasteHeat_power/1
  [hvs_API1_wasteHeat_power] -> Sum8/1
  [hvs_API3_wasteHeat_power] -> Sum8/2
  [hvs_DCL_wasteHeat_power] -> Sum8/3
  [hvs_dcdc_current] -> DC_Link/3
  Reshape/1 -> hvs_dcLink_electricalEnergyStorage_current/1
  Reshape1/1 -> [hvs_dcdcConverter_voltage]
  Reshape2/1 -> [hvs_inverter_BrakeResistor_voltage]
  Reshape3/1 -> [hvs_inverter_drive_emot_voltage]
  Reshape4/1 -> [hvs_charger_DCLink_vlt]
  Reshape5/1 -> [hvs_APIs_DCLink_vlt]
  Reshape7/1 -> hvs_BRC_ACT_DcLinkVoltage/1
  Reshape8/1 -> PTI_DriveEmot_Bosch_10ms/1
  Reshape10/1 -> hvs_EMD4_ACT_DcLinkVoltage/1
  Reshape11/1 -> Charger/5
  Reshape12/1 -> hvs_VCCU_DCLInk_vlt/1
  [dcLink_aux_current] -> DC_Link/10
  env_dcLink_aux_power/1 -> [dcLink_aux_power], sub_env_aux/1(env_dcLink_aux_power)
  sub_env_aux/1(dcLink_aux_current) -> [dcLink_aux_current]
  [hvs_dcLink_electricalEnergyStorage_voltage] -> sub_env_aux/2(Nebenagg_voltage)
  DC_Link/8 -> Reshape15/1
  hvsAux_dcdcConverter_LvVoltage_Rq/1 -> Process/6(hvsAux_dcdcConv_LvVoltage_Rq), DC_DC/4  "hvsAux_dcdcConverter_LvVoltage_Rq"
  Charger/1 -> hvs_DCBoxWasteHeat_power/1  "hvs_DCBoxWasteHeat_power"
  hvs_DCBoxCoolant_Temperature/1 -> Terminator4/1
  env_Temperature/1 -> ePTO_MODEL/1, [env_Temperature]
  Reshape17/1 -> [hvs_ePTO_DCLink_vlt]
  DC_Link/10 -> Reshape17/1
  ePTO_MODEL/1 -> [hvs_dcLink_ePTO_current]
  ePTO_MODEL/2 -> hvs_ePTO_Elec_Power/1
  ePTO_MODEL/3 -> Terminator7/1
  [hvs_APIs_DCLink_vlt] -> ePTO_MODEL/2
  [hvs_dcLink_ePTO_current] -> DC_Link/12
  [hvs_dcdc_current] -> Process/2(hvs_dcdc_HvCurrent)  "hvs_dcdc_HvCurrent"
  hvs_drvEmotCoolant_Temperature/1 -> Process/3(hvs_drvEmotCoolant_Temperature)
  [dcLink_aux_power] -> Process/4(dcLink_aux_power)  "dcLink_aux_power"
  hvs_dcdcConverter_current/1 -> Process/5(hvs_dcdcConv_current)
  Process/1(dcdc_conv_eff) -> DC_DC/2
  Process/2(hvs_dcdcConv_current1) -> DC_DC/3
  hvs_emot_Emot3_angAcc/1 -> Terminator6/1
  hvs_emot_Emot3_angPos/1 -> Terminator8/1
  hvs_emot_Emot4_angAcc/1 -> Terminator9/1
  hvs_emot_Emot4_angPos/1 -> Terminator10/1
  hvs_emot_Emot4_angVel/1 -> rad/sectorpm3/1
  hvs_emot_Emot3_angVel/1 -> rad/sectorpm2/1
  PTI_DriveEmot_Bosch_10ms/12 -> hvs_EMD1_ACT_DigitalInput1/1
  PTI_DriveEmot_Bosch_10ms/1 -> [hvs_dcLink_drive_emot_current]
  PTI_DriveEmot_Bosch_10ms/4 -> hvs_emot_Emot3_torque/1
  PTI_DriveEmot_Bosch_10ms/5 -> hvs_emot_Emot4_torque/1
  PTI_DriveEmot_Bosch_10ms/8 -> hvs_drvEmot1WasteHeat_power/1
  PTI_DriveEmot_Bosch_10ms/9 -> hvs_drvEmot2WasteHeat_power/1
  PTI_DriveEmot_Bosch_10ms/10 -> hvs_drvEmot3WasteHeat_power/1
  PTI_DriveEmot_Bosch_10ms/11 -> hvs_drvEmot4WasteHeat_power/1
  [hvs_dcLink_drive_emot_current] -> hvs_dcLink_drive_emot_current/1
  [hvs_dcLink_BrakeResistor_current] -> hvs_dcLink_BrakeResistor_current/1
  [env_Temperature] -> PTI_DriveEmot_Bosch_10ms/40
  hvs_drvEmot3Coolant_Temperature/1 -> Rename_Signals_for_PTI_detailed/3(hvs_drvEmot3Coolant_Temperature), PTI_DriveEmot_Bosch_10ms/39
  hvs_drvEmot3Oil_Temperature/1 -> PTI_DriveEmot_Bosch_10ms/38
  hvs_drvEmot2Oil_Temperature/1 -> PTI_DriveEmot_Bosch_10ms/36
  hvs_drvEmot4Coolant_Temperature/1 -> Rename_Signals_for_PTI_detailed/4(hvs_drvEmot4Coolant_Temperature), PTI_DriveEmot_Bosch_10ms/35
  hvs_drvEmot4Oil_Temperature/1 -> PTI_DriveEmot_Bosch_10ms/34
  hvs_drvEmot1Coolant_Temperature/1 -> Rename_Signals_for_PTI_detailed/1(hvs_drvEmot1Coolant_Temperature), PTI_DriveEmot_Bosch_10ms/33
  hvs_drvEmot1Oil_Temperature/1 -> PTI_DriveEmot_Bosch_10ms/32
  hvs_driveInverter_coolant_temperature/1 -> PTI_DriveEmot_Bosch_10ms/31
  rad/sectorpm/1 -> PTI_DriveEmot_Bosch_10ms/27
  rad/sectorpm1/1 -> PTI_DriveEmot_Bosch_10ms/28
  rad/sectorpm2/1 -> PTI_DriveEmot_Bosch_10ms/29
  rad/sectorpm3/1 -> PTI_DriveEmot_Bosch_10ms/30
  pti_frqSwt_PTI2/1 -> PTI_DriveEmot_Bosch_10ms/24
  pti_frqSwt_PTI3/1 -> PTI_DriveEmot_Bosch_10ms/25
  pti_frqSwt_PTI4/1 -> PTI_DriveEmot_Bosch_10ms/26
  hvs_drvEmot1CoolantFlow_vdot/1 -> PTI_DriveEmot_Bosch_10ms/41
  hvs_drvEmot1OilFlow_vdot/1 -> PTI_DriveEmot_Bosch_10ms/42
  hvs_driveInverterCoolantFlow_vdot/1 -> PTI_DriveEmot_Bosch_10ms/43
  hvs_drvEmot3OilFlow_vdot/1 -> PTI_DriveEmot_Bosch_10ms/49
  hvs_drvEmot3CoolantFlow_vdot/1 -> PTI_DriveEmot_Bosch_10ms/48
  hvs_drvEmot2OilFlow_vdot/1 -> PTI_DriveEmot_Bosch_10ms/47
  hvs_drvEmot2CoolantFlow_vdot/1 -> PTI_DriveEmot_Bosch_10ms/46
  hvs_drvEmot4OilFlow_vdot/1 -> PTI_DriveEmot_Bosch_10ms/45
  hvs_drvEmot4CoolantFlow_vdot/1 -> PTI_DriveEmot_Bosch_10ms/44
  PTI_DriveEmot_Bosch_10ms/120 -> hvs_EMD2_ACT_Torque_Nm/1
  PTI_DriveEmot_Bosch_10ms/122 -> hvs_EMD1_ACT_Torque_Nm/1
  PTI_DriveEmot_Bosch_10ms/121 -> hvs_EMD3_ACT_Torque_Nm/1
  PTI_DriveEmot_Bosch_10ms/123 -> hvs_EMD4_ACT_Torque_Nm/1
  PTI_DriveEmot_Bosch_10ms/124 -> hvs_drvEmot2WasteHeatcoolant_power/1
  PTI_DriveEmot_Bosch_10ms/125 -> hvs_drvEmot2WasteHeatoil_power/1
  PTI_DriveEmot_Bosch_10ms/126 -> hvs_drvEmot3WasteHeatcoolant_power/1
  PTI_DriveEmot_Bosch_10ms/127 -> hvs_drvEmot3WasteHeatoil_power/1
  PTI_DriveEmot_Bosch_10ms/128 -> hvs_drvEmot1WasteHeatcoolant_power/1
  PTI_DriveEmot_Bosch_10ms/129 -> hvs_drvEmot1WasteHeatoil_power/1
  PTI_DriveEmot_Bosch_10ms/130 -> hvs_drvEmot4WasteHeatcoolant_power/1
  PTI_DriveEmot_Bosch_10ms/131 -> hvs_drvEmot4WasteHeatoil_power/1
  brc_ControlMode/1 -> Brake Chopper RX1/1
  brc_PowerReqCh1_kW/1 -> Brake Chopper RX1/2
  brc_PowerReqCh2_kW/1 -> Brake Chopper RX1/3
  Reshape6/1 -> Brake Chopper RX1/4
  hvs_brakeResistor_coolant_temperature/1 -> Brake Chopper RX1/6
  Brake Chopper RX1/1 -> hvs_BRC_ACT_DigitalInput1/1
  Brake Chopper RX1/2 -> hvs_BRC_ACT_InverterState/1
  Brake Chopper RX1/3 -> hvs_BRC_ACT_MaxAvailablePowerCh1/1
  Brake Chopper RX1/4 -> hvs_BRC_ACT_MaxAvailablePowerCh1_VAL/1
  Brake Chopper RX1/5 -> hvs_BRC_ACT_PowerCh1/1
  Brake Chopper RX1/6 -> hvs_BRC_ACT_MaxAvailablePowerCh2/1
  Brake Chopper RX1/7 -> hvs_BRC_ACT_PowerCh2/1
  Brake Chopper RX1/8 -> Reshape7/1
  Brake Chopper RX1/9 -> hvs_BRC_ACT_ExtTemperatureCh1/1
  Brake Chopper RX1/10 -> hvs_BRC_ACT_ExtTemperatureCh2/1
  Brake Chopper RX1/11 -> hvs_BRC_ACT_JunctionTempCh1/1
  Brake Chopper RX1/12 -> hvs_BRC_ACT_JunctionTempCh2/1
  Brake Chopper RX1/13 -> hvs_brakeResistor_wasteHeat_power/1
  Brake Chopper RX1/14 -> [hvs_dcLink_BrakeResistor_current]
  Brake Chopper RX1/15 -> hvs_BRC_ACT_MaxAvailablePowerCh1_kW/1
  Brake Chopper RX1/16 -> hvs_BRC_ACT_PowerCh1_kW/1
  Brake Chopper RX1/17 -> hvs_BRC_ACT_MaxAvailablePowerCh2_kW/1
  Brake Chopper RX1/18 -> hvs_BRC_ACT_PowerCh2_kW/1

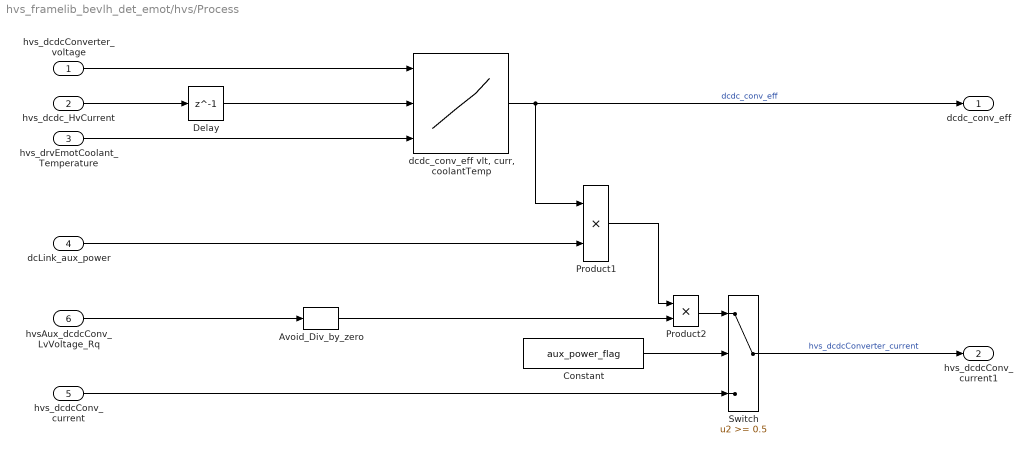
== system hvs_framelib_bevlh_det_emot/hvs/Process ==
  hvs_dcdcConverter_voltage : Inport
  hvs_dcdc_HvCurrent : Inport  Port=2
  hvs_drvEmotCoolant_Temperature : Inport  Port=3
  dcLink_aux_power : Inport  Port=4
  hvs_dcdcConv_current : Inport  Port=5
  hvsAux_dcdcConv_LvVoltage_Rq : Inport  Port=6
  Avoid_Div_by_zero : Electrical_converter/DC_DC/Avoid_Div_by_zero
  Constant : Constant  Value=aux_power_flag
  Delay : Delay  DelayLength=1  InitialCondition=0
  Product1 : Product  Inputs=**  RndMeth=Zero
  Product2 : Product  Inputs=**  RndMeth=Zero
  Switch : Switch  Threshold=0.5
  "dcdc_conv_eff vlt, curr, coolantTemp" : Lookup_n-D  NumberOfTableDimensions=3  BreakpointsForDimension1=dcdc_effmap_vlt_1stD  BreakpointsForDimension2=dcdc_effmap_cur_2ndD  BreakpointsForDimension3=dcdc_effmap_cooltemp_3rdD  Table=dcdc_effmap  ExtrapMethod=Clip  RndMeth=Simplest  InputSameDT=on
  dcdc_conv_eff : Outport
  hvs_dcdcConv_current1 : Outport  Port=2
  wires:
  Delay/1 -> "dcdc_conv_eff vlt, curr, coolantTemp"/2
  hvs_dcdc_HvCurrent/1 -> Delay/1
  "dcdc_conv_eff vlt, curr, coolantTemp"/1 -> dcdc_conv_eff/1, Product1/1  "dcdc_conv_eff"
  Product2/1 -> Switch/1
  Product1/1 -> Product2/1
  hvs_dcdcConv_current/1 -> Switch/3
  Switch/1 -> hvs_dcdcConv_current1/1  "hvs_dcdcConverter_current"
  dcLink_aux_power/1 -> Product1/2
  Avoid_Div_by_zero/1 -> Product2/2
  Constant/1 -> Switch/2
  hvsAux_dcdcConv_LvVoltage_Rq/1 -> Avoid_Div_by_zero/1
  hvs_dcdcConverter_voltage/1 -> "dcdc_conv_eff vlt, curr, coolantTemp"/1
  hvs_drvEmotCoolant_Temperature/1 -> "dcdc_conv_eff vlt, curr, coolantTemp"/3

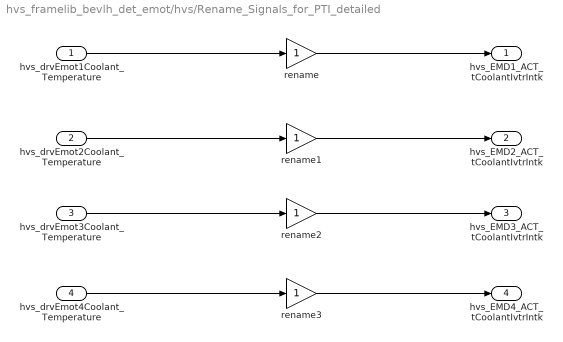
== system hvs_framelib_bevlh_det_emot/hvs/Rename_Signals_for_PTI_detailed ==
  hvs_drvEmot1Coolant_Temperature : Inport
  hvs_drvEmot2Coolant_Temperature : Inport  Port=2
  hvs_drvEmot3Coolant_Temperature : Inport  Port=3
  hvs_drvEmot4Coolant_Temperature : Inport  Port=4
  rename{,1..3} (4 alike) : Gain
  hvs_EMD1_ACT_tCoolantIvtrIntk : Outport
  hvs_EMD2_ACT_tCoolantIvtrIntk : Outport  Port=2
  hvs_EMD3_ACT_tCoolantIvtrIntk : Outport  Port=3
  hvs_EMD4_ACT_tCoolantIvtrIntk : Outport  Port=4
  wires:
  hvs_drvEmot1Coolant_Temperature/1 -> rename/1
  rename/1 -> hvs_EMD1_ACT_tCoolantIvtrIntk/1
  hvs_drvEmot4Coolant_Temperature/1 -> rename3/1
  hvs_drvEmot3Coolant_Temperature/1 -> rename2/1
  hvs_drvEmot2Coolant_Temperature/1 -> rename1/1
  rename1/1 -> hvs_EMD2_ACT_tCoolantIvtrIntk/1
  rename2/1 -> hvs_EMD3_ACT_tCoolantIvtrIntk/1
  rename3/1 -> hvs_EMD4_ACT_tCoolantIvtrIntk/1

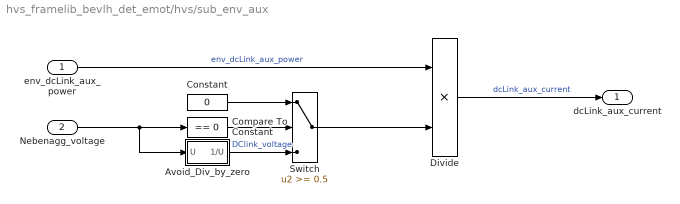
== system hvs_framelib_bevlh_det_emot/hvs/sub_env_aux ==
  env_dcLink_aux_power : Inport
  Nebenagg_voltage : Inport  Port=2
  Avoid_Div_by_zero : Subsystem
  Compare To Constant : simulink/Logic and Bit Operations/Compare To Constant  relop===  const=0  OutDataTypeStr=boolean
  Constant : Constant  Value=0
  Divide : Product
  Switch : Switch  Threshold=0.5
  dcLink_aux_current : Outport
  wires:
  Divide/1 -> dcLink_aux_current/1  "dcLink_aux_current"
  Nebenagg_voltage/1 -> Avoid_Div_by_zero/1(U), Compare To Constant/1
  Avoid_Div_by_zero/1(1/U) -> Switch/3  "DClink_voltage"
  env_dcLink_aux_power/1 -> Divide/1  "env_dcLink_aux_power"
  Compare To Constant/1 -> Switch/2
  Constant/1 -> Switch/1
  Switch/1 -> Divide/2

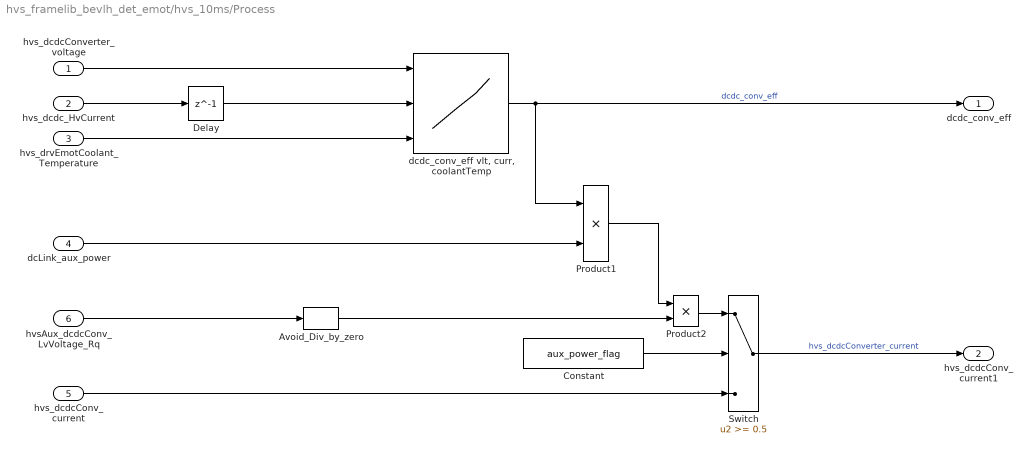
== system hvs_framelib_bevlh_det_emot/hvs_10ms/Process ==
  hvs_dcdcConverter_voltage : Inport
  hvs_dcdc_HvCurrent : Inport  Port=2
  hvs_drvEmotCoolant_Temperature : Inport  Port=3
  dcLink_aux_power : Inport  Port=4
  hvs_dcdcConv_current : Inport  Port=5
  hvsAux_dcdcConv_LvVoltage_Rq : Inport  Port=6
  Avoid_Div_by_zero : Electrical_converter/DC_DC/Avoid_Div_by_zero
  Constant : Constant  Value=aux_power_flag
  Delay : Delay  DelayLength=1  InitialCondition=0
  Product1 : Product  Inputs=**  RndMeth=Zero
  Product2 : Product  Inputs=**  RndMeth=Zero
  Switch : Switch  Threshold=0.5
  "dcdc_conv_eff vlt, curr, coolantTemp" : Lookup_n-D  NumberOfTableDimensions=3  BreakpointsForDimension1=dcdc_effmap_vlt_1stD  BreakpointsForDimension2=dcdc_effmap_cur_2ndD  BreakpointsForDimension3=dcdc_effmap_cooltemp_3rdD  Table=dcdc_effmap  ExtrapMethod=Clip  RndMeth=Simplest  InputSameDT=on
  dcdc_conv_eff : Outport
  hvs_dcdcConv_current1 : Outport  Port=2
  wires:
  hvs_drvEmotCoolant_Temperature/1 -> "dcdc_conv_eff vlt, curr, coolantTemp"/3
  hvs_dcdcConverter_voltage/1 -> "dcdc_conv_eff vlt, curr, coolantTemp"/1
  hvsAux_dcdcConv_LvVoltage_Rq/1 -> Avoid_Div_by_zero/1
  Constant/1 -> Switch/2
  Avoid_Div_by_zero/1 -> Product2/2
  dcLink_aux_power/1 -> Product1/2
  Switch/1 -> hvs_dcdcConv_current1/1  "hvs_dcdcConverter_current"
  hvs_dcdcConv_current/1 -> Switch/3
  Product1/1 -> Product2/1
  Product2/1 -> Switch/1
  "dcdc_conv_eff vlt, curr, coolantTemp"/1 -> Product1/1, dcdc_conv_eff/1  "dcdc_conv_eff"
  hvs_dcdc_HvCurrent/1 -> Delay/1
  Delay/1 -> "dcdc_conv_eff vlt, curr, coolantTemp"/2

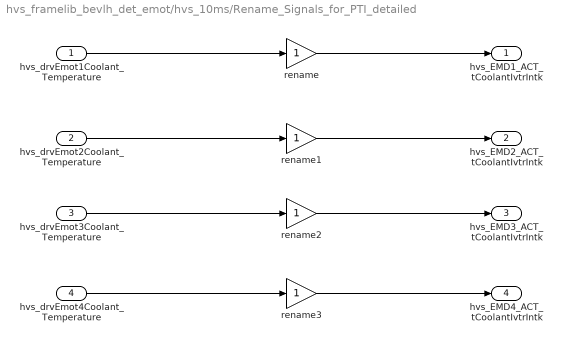
== system hvs_framelib_bevlh_det_emot/hvs_10ms/Rename_Signals_for_PTI_detailed ==
  hvs_drvEmot1Coolant_Temperature : Inport
  hvs_drvEmot2Coolant_Temperature : Inport  Port=2
  hvs_drvEmot3Coolant_Temperature : Inport  Port=3
  hvs_drvEmot4Coolant_Temperature : Inport  Port=4
  rename{,1..3} (4 alike) : Gain
  hvs_EMD1_ACT_tCoolantIvtrIntk : Outport
  hvs_EMD2_ACT_tCoolantIvtrIntk : Outport  Port=2
  hvs_EMD3_ACT_tCoolantIvtrIntk : Outport  Port=3
  hvs_EMD4_ACT_tCoolantIvtrIntk : Outport  Port=4
  wires:
  rename3/1 -> hvs_EMD4_ACT_tCoolantIvtrIntk/1
  rename2/1 -> hvs_EMD3_ACT_tCoolantIvtrIntk/1
  rename1/1 -> hvs_EMD2_ACT_tCoolantIvtrIntk/1
  hvs_drvEmot2Coolant_Temperature/1 -> rename1/1
  hvs_drvEmot3Coolant_Temperature/1 -> rename2/1
  hvs_drvEmot4Coolant_Temperature/1 -> rename3/1
  rename/1 -> hvs_EMD1_ACT_tCoolantIvtrIntk/1
  hvs_drvEmot1Coolant_Temperature/1 -> rename/1

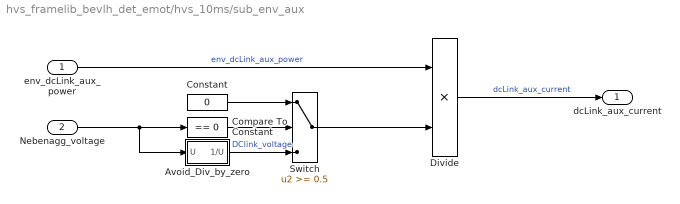
== system hvs_framelib_bevlh_det_emot/hvs_10ms/sub_env_aux ==
  env_dcLink_aux_power : Inport
  Nebenagg_voltage : Inport  Port=2
  Avoid_Div_by_zero : Subsystem
  Compare To Constant : simulink/Logic and Bit Operations/Compare To Constant  relop===  const=0  OutDataTypeStr=boolean
  Constant : Constant  Value=0
  Divide : Product
  Switch : Switch  Threshold=0.5
  dcLink_aux_current : Outport
  wires:
  Switch/1 -> Divide/2
  Constant/1 -> Switch/1
  Compare To Constant/1 -> Switch/2
  env_dcLink_aux_power/1 -> Divide/1  "env_dcLink_aux_power"
  Avoid_Div_by_zero/1(1/U) -> Switch/3  "DClink_voltage"
  Nebenagg_voltage/1 -> Compare To Constant/1, Avoid_Div_by_zero/1(U)
  Divide/1 -> dcLink_aux_current/1  "dcLink_aux_current"

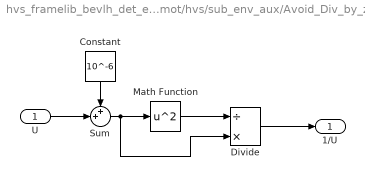
== system hvs_framelib_bevlh_det_emot/hvs/sub_env_aux/Avoid_Div_by_zero ==
  U : Inport
  Constant : Constant  Value=10^-6
  Divide : Product  Inputs=/*
  Math Function : Math  Operator=square  SaturateOnIntegerOverflow=on
  Sum : Sum  Inputs=++|
  1/U : Outport
  wires:
  U/1 -> Sum/2
  Constant/1 -> Sum/1
  Sum/1 -> Math Function/1, Divide/2
  Math Function/1 -> Divide/1
  Divide/1 -> 1/U/1

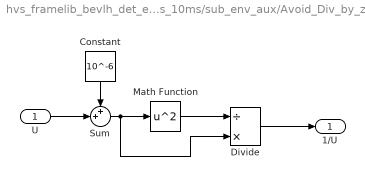
== system hvs_framelib_bevlh_det_emot/hvs_10ms/sub_env_aux/Avoid_Div_by_zero ==
  U : Inport
  Constant : Constant  Value=10^-6
  Divide : Product  Inputs=/*
  Math Function : Math  Operator=square  SaturateOnIntegerOverflow=on
  Sum : Sum  Inputs=++|
  1/U : Outport
  wires:
  Divide/1 -> 1/U/1
  Math Function/1 -> Divide/1
  Sum/1 -> Divide/2, Math Function/1
  Constant/1 -> Sum/1
  U/1 -> Sum/2
